simulink model "iterative_motion_controller"  (R2023b)
settings: Solver=FixedStepDiscrete  StartTime=0.0  StopTime=1  RelTol=1e-3
undefined symbols (not defined in the file): InitConfParams
settings Model: DataDictionary=amcfoc.sldd  Creator=mfussi  LastModifiedBy=mfussi
settings SolverCC: ConcurrentTasks=on  AutoInsertRateTranBlk=on  InsertRTBMode=Never (minimum delay)
settings DataIOCC: SaveOutput=off  SignalLogging=off  DSMLogging=off  SaveTime=off  ReturnWorkspaceOutputs=off
settings OptimizationCC: DefaultParameterBehavior=Inlined  UseDivisionForNetSlopeComputation=on  GainParamInheritBuiltInType=on  UseFloatMulNetSlope=on  DefaultUnderspecifiedDataType=single  UseSpecifiedMinMax=on  InlineInvariantSignals=on  PassReuseOutputArgsAs=Individual arguments  ZeroExternalMemoryAtStartup=off  ZeroInternalMemoryAtStartup=off  SimCompilerOptimization=on  OptimizeBlockOrder=speed  DifferentSizesBufferReuse=on  EfficientTunableParamExpr=on
settings DebuggingCC: ParameterTunabilityLossMsg=error
settings HardwareCC: ProdBitPerPointer=32  ProdBitPerSizeT=32  ProdBitPerPtrDiffT=32  ProdLargestAtomicInteger=Long  ProdLargestAtomicFloat=Double  ProdWordSize=32  ProdLongLongMode=on  ProdHWDeviceType=ARM Compatible->ARM Cortex-M
settings ModelReferenceCC: UpdateModelReferenceTargets=Force
settings SFSimCC: MATLABDynamicMemAlloc=off
settings RTWCC: Description=Embedded Coder  SystemTargetFile=ert.tlc  GenCodeOnly=on  PackageGeneratedCodeAndArtifacts=on  TemplateMakefile=ert_default_tmf  Toolchain=GNU Tools for ARM Embedded Processors  BuildConfiguration=Faster Runs
settings CodeAppCC: ForceParamTrailComments=on  IgnoreCustomStorageClasses=off  MaxIdLength=60  OperatorAnnotations=on  SimulinkDataObjDesc=on  SFDataObjDesc=on  InsertBlockDesc=on
settings ERTTargetCC: TargetLangStandard=C99 (ISO)  CodeReplacementLibrary=ARM Cortex-M,iCubTech  GenerateSampleERTMain=on  CombineSignalStateStructs=on  SuppressErrorStatus=on  SupportNonFinite=off  InlinedParameterPlacement=NonHierarchical  RootIOFormat=Structure reference  ERTCustomFileTemplate=example_file_process.tlc

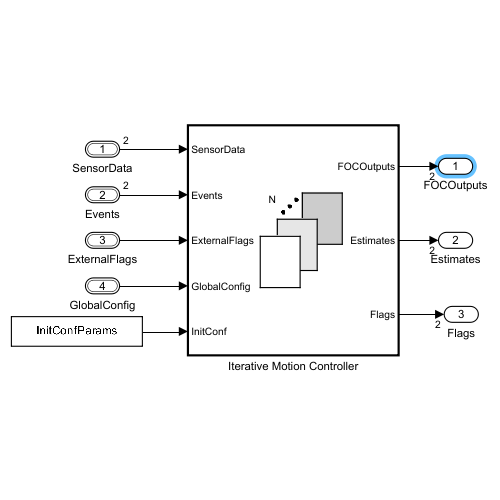
[thumbnail: Simulink's stored preview of the top-level diagram]
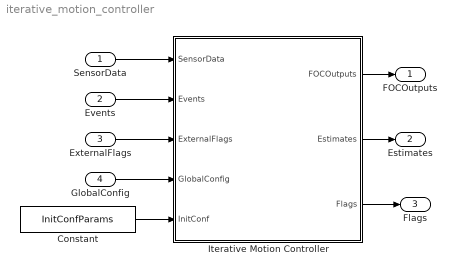
== system iterative_motion_controller ==
  SensorData : Inport  OutDataTypeStr=Bus: SensorsData  PortDimensions=numberOfActuators  BusOutputAsStruct=on
  Events : Inport  Port=2  OutDataTypeStr=Bus: SupervisorReceivedEvents  PortDimensions=numberOfActuators  BusOutputAsStruct=on
  ExternalFlags : Inport  Port=3  OutDataTypeStr=Bus: ExternalFlags  BusOutputAsStruct=on
  GlobalConfig : Inport  Port=4  OutDataTypeStr=Bus: GlobalConfiguration  BusOutputAsStruct=on
  Constant : Constant  Value=InitConfParams  OutDataTypeStr=Bus: ActuatorConfiguration  SampleTime=1e-3
  Iterative Motion Controller : Subsystem  TreatAsAtomicUnit=on
  FOCOutputs : Outport  PortDimensions=numberOfActuators
  Estimates : Outport  Port=2  PortDimensions=numberOfActuators
  Flags : Outport  Port=3  PortDimensions=numberOfActuators
  wires:
  SensorData/1 -> Iterative Motion Controller/1(SensorData)
  Iterative Motion Controller/1(FOCOutputs) -> FOCOutputs/1
  Iterative Motion Controller/2(Estimates) -> Estimates/1
  Events/1 -> Iterative Motion Controller/2(Events)
  ExternalFlags/1 -> Iterative Motion Controller/3(ExternalFlags)
  GlobalConfig/1 -> Iterative Motion Controller/4(GlobalConfig)
  Constant/1 -> Iterative Motion Controller/5(InitConf)
  Iterative Motion Controller/3(Flags) -> Flags/1

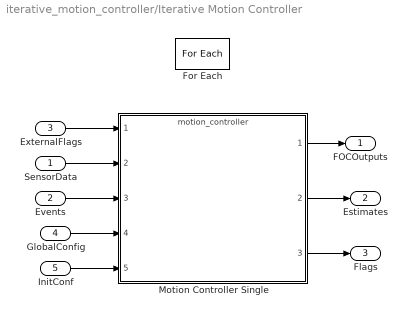
== system iterative_motion_controller/Iterative Motion Controller ==
  SensorData : Inport  OutDataTypeStr=Bus: SensorsData  Partition=on  PartitionDimension=1  PartitionWidth=1  PartitionOffset=0
  Events : Inport  Port=2  OutDataTypeStr=Bus: SupervisorReceivedEvents  Partition=on  PartitionDimension=1  PartitionWidth=1  PartitionOffset=0
  ExternalFlags : Inport  Port=3  OutDataTypeStr=Bus: ExternalFlags
  GlobalConfig : Inport  Port=4  OutDataTypeStr=Bus: GlobalConfiguration
  InitConf : Inport  Port=5  OutDataTypeStr=Bus: ActuatorConfiguration  Partition=on  PartitionDimension=1  PartitionWidth=1  PartitionOffset=0
  For Each : ForEach  DisableCoverage=on
  Motion Controller Single : ModelReference  ModelNameDialog=motion_controller.slx  ModelReferenceVersion=2.190
  FOCOutputs : Outport  OutDataTypeStr=Bus: FOCOutputs  ConcatenationDimension=1
  Estimates : Outport  Port=2  OutDataTypeStr=Bus: EstimatedData  ConcatenationDimension=1
  Flags : Outport  Port=3  OutDataTypeStr=Bus: Flags  ConcatenationDimension=1
  wires:
  SensorData/1 -> Motion Controller Single/2
  Events/1 -> Motion Controller Single/3
  ExternalFlags/1 -> Motion Controller Single/1
  GlobalConfig/1 -> Motion Controller Single/4
  Motion Controller Single/1 -> FOCOutputs/1
  Motion Controller Single/2 -> Estimates/1
  InitConf/1 -> Motion Controller Single/5
  Motion Controller Single/3 -> Flags/1
